simulink model "navigator"  (R2013b)
settings: Solver=FixedStepDiscrete  StartTime=0.0  StopTime=inf  FixedStep=0.1  RelTol=1e-3
undefined symbols (not defined in the file): Earth, WGS84
libraries: aerolibtransform2 x3, simulink_extras x2
settings Model: Creator=Matteo  LastModifiedBy=Gianluca Rossetti
settings OptimizationCC: OptimizeModelRefInitCode=on  LifeSpan=Inf
settings HardwareCC: ProdBitPerInt=16  ProdBitPerPointer=8  ProdIntDivRoundTo=Zero  ProdEndianess=LittleEndian  ProdWordSize=8  ProdHWDeviceType=Atmel->AVR
settings RTWCC: SystemTargetFile=ert.tlc  GenCodeOnly=on  TemplateMakefile=ert_default_tmf  Description=Embedded Coder  ProcessScript=ert_make_rtw_hook  BuildConfiguration=Faster Runs  TargetLang=C++  CheckMdlBeforeBuild=Warning
settings CodeAppCC: IgnoreCustomStorageClasses=off
settings ERTTargetCC: CodeReplacementLibrary=ANSI_C  GenerateSampleERTMain=on  ERTCustomFileTemplate=example_file_process.tlc

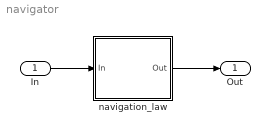
== system navigator ==
  In : Inport  OutDataTypeStr=single  PortDimensions=16
  navigation_law : Subsystem
  Out : Outport  OutDataTypeStr=single  PortDimensions=8
  wires:
  In/1 -> navigation_law/1(In)
  navigation_law/1(Out) -> Out/1

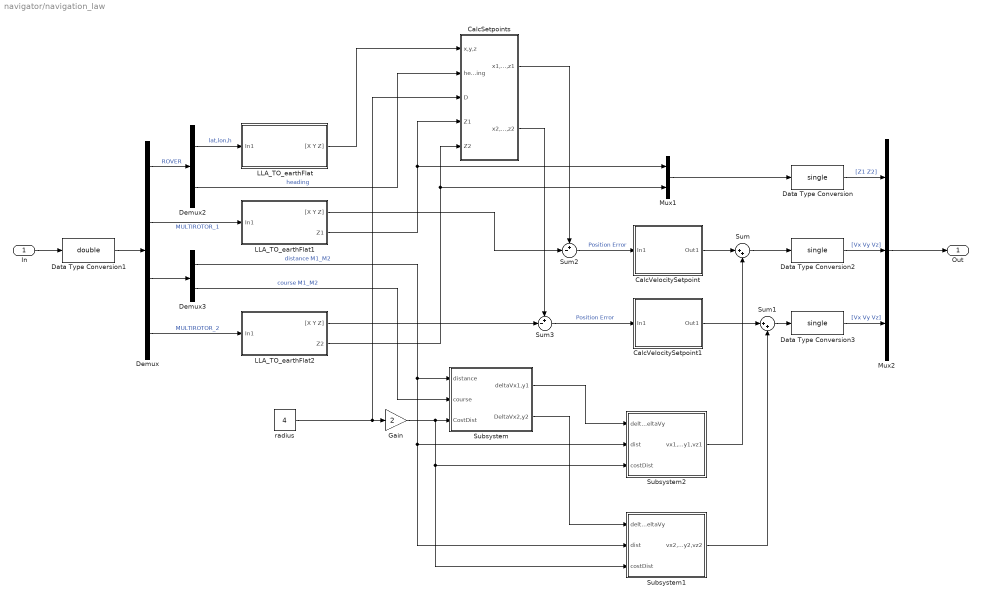
== system navigator/navigation_law ==
  In : Inport
  CalcSetpoints : Subsystem
  CalcVelocitySetpoint : Subsystem
  CalcVelocitySetpoint1 : Subsystem
  Data Type Conversion : DataTypeConversion  OutDataTypeStr=single
  Data Type Conversion1 : DataTypeConversion  OutDataTypeStr=double
  Data Type Conversion2 : DataTypeConversion  OutDataTypeStr=single
  Data Type Conversion3 : DataTypeConversion  OutDataTypeStr=single
  Demux : Demux  Outputs=[4 5 2 5]
  Demux2 : Demux  Outputs=[3 1]
  Demux3 : Demux  Outputs=2
  Gain : Gain  Gain=2
  LLA_TO_earthFlat : Subsystem
  LLA_TO_earthFlat1 : Subsystem
  LLA_TO_earthFlat2 : Subsystem
  Mux1 : Mux  Inputs=[1 1]
  Mux2 : Mux  Inputs=[2 3 3]
  Subsystem : Subsystem
  Subsystem1 : Subsystem
  Subsystem2 : Subsystem
  Sum : Sum  Inputs=|++
  Sum1 : Sum  Inputs=|++
  Sum2 : Sum  Inputs=+-|
  Sum3 : Sum  Inputs=+-|
  radius : Constant  Value=4
  Out : Outport
  wires:
  Demux/1 -> Demux2/1  "ROVER"
  Demux/4 -> LLA_TO_earthFlat2/1(In1)  "MULTIROTOR_2"
  Data Type Conversion/1 -> Mux2/1  "[Z1 Z2]"
  In/1 -> Data Type Conversion1/1
  Data Type Conversion1/1 -> Demux/1
  Mux2/1 -> Out/1
  Demux/2 -> LLA_TO_earthFlat1/1(In1)  "MULTIROTOR_1"
  LLA_TO_earthFlat1/1("[X Y Z]") -> Sum2/2
  Data Type Conversion2/1 -> Mux2/2  "[Vx Vy Vz]"
  Sum2/1 -> CalcVelocitySetpoint/1(In1)  "Position Error"
  CalcVelocitySetpoint/1(Out1) -> Sum/1
  LLA_TO_earthFlat2/1("[X Y Z]") -> Sum3/2
  Sum3/1 -> CalcVelocitySetpoint1/1(In1)  "Position Error"
  CalcVelocitySetpoint1/1(Out1) -> Sum1/1
  Data Type Conversion3/1 -> Mux2/3  "[Vx Vy Vz]"
  Demux2/1 -> LLA_TO_earthFlat/1(In1)  "lat,lon,h"
  LLA_TO_earthFlat/1("[X Y Z]") -> CalcSetpoints/1(x,y,z)
  Demux2/2 -> CalcSetpoints/2(heading)  "heading"
  CalcSetpoints/1(x1,y1,z1) -> Sum2/1
  CalcSetpoints/2(x2,y2,z2) -> Sum3/1
  radius/1 -> Gain/1, CalcSetpoints/3(D)
  LLA_TO_earthFlat1/2(Z1) -> Mux1/1, CalcSetpoints/4(Z1)
  LLA_TO_earthFlat2/2(Z2) -> CalcSetpoints/5(Z2), Mux1/2
  Demux/3 -> Demux3/1
  Demux3/1 -> Subsystem1/2(dist), Subsystem2/2(dist), Subsystem/1(distance)  "distance M1_M2"
  Sum/1 -> Data Type Conversion2/1
  Sum1/1 -> Data Type Conversion3/1
  Subsystem/1(deltaVx1,y1) -> Subsystem2/1("deltaVx, deltaVy")
  Mux1/1 -> Data Type Conversion/1
  Demux3/2 -> Subsystem/2(course)  "course M1_M2"
  Subsystem/2(DeltaVx2,y2) -> Subsystem1/1("deltaVx, deltaVy")
  Subsystem1/1(vx2,vy2,vz2) -> Sum1/2
  Subsystem2/1(vx1,vy1,vz1) -> Sum/2
  Gain/1 -> Subsystem1/3(costDist), Subsystem2/3(costDist), Subsystem/3(CostDist)

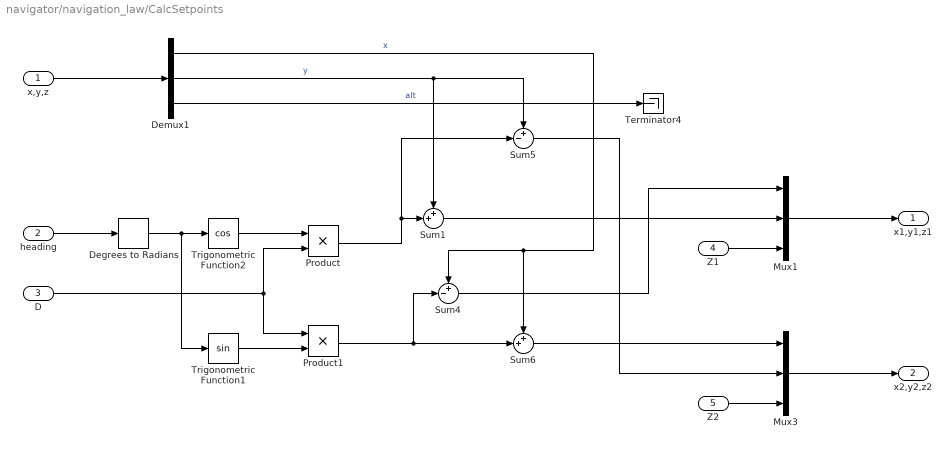
== system navigator/navigation_law/CalcSetpoints ==
  x,y,z : Inport
  heading : Inport  Port=2
  D : Inport  Port=3
  Z1 : Inport  Port=4
  Z2 : Inport  Port=5
  Degrees to Radians : simulink_extras/Transformations/Degrees to Radians
  Demux1 : Demux  Outputs=[1 1 1]
  Mux1 : Mux  Inputs=[1 1 1]
  Mux3 : Mux  Inputs=[1 1 1]
  Product : Product
  Product1 : Product
  Sum1 : Sum  Inputs=++|
  Sum4 : Sum  Inputs=+-|
  Sum5 : Sum  Inputs=+-|
  Sum6 : Sum  Inputs=++|
  Terminator4 : Terminator
  Trigonometric Function1 : Trigonometry
  Trigonometric Function2 : Trigonometry  Operator=cos
  x1,y1,z1 : Outport
  x2,y2,z2 : Outport  Port=2
  wires:
  Sum5/1 -> Mux3/2
  Sum6/1 -> Mux3/1
  Mux3/1 -> x2,y2,z2/1
  Demux1/1 -> Sum4/1, Sum6/1  "x"
  Mux1/1 -> x1,y1,z1/1
  Sum4/1 -> Mux1/1
  Product1/1 -> Sum6/2, Sum4/2
  heading/1 -> Degrees to Radians/1
  Demux1/2 -> Sum5/1, Sum1/1  "y"
  Sum1/1 -> Mux1/2
  Demux1/3 -> Terminator4/1  "alt"
  Product/1 -> Sum5/2, Sum1/2
  D/1 -> Product1/1, Product/2
  x,y,z/1 -> Demux1/1
  Degrees to Radians/1 -> Trigonometric Function1/1, Trigonometric Function2/1
  Trigonometric Function2/1 -> Product/1
  Trigonometric Function1/1 -> Product1/2
  Z2/1 -> Mux3/3
  Z1/1 -> Mux1/3

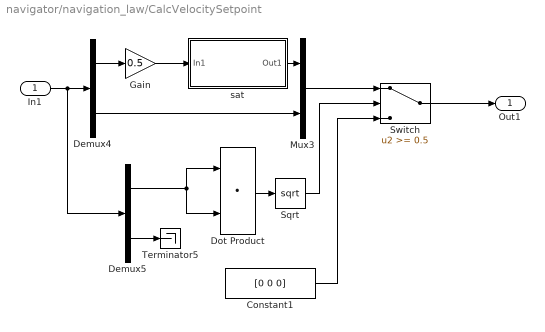
== system navigator/navigation_law/CalcVelocitySetpoint ==
  In1 : Inport
  Constant1 : Constant  Value=[0 0 0]
  Demux4 : Demux  Outputs=[2 1]
  Demux5 : Demux  Outputs=[2 1]
  Dot Product : DotProduct  InputSameDT=on  OutDataTypeStr=Inherit: Inherit via internal rule
  Gain : Gain  Gain=0.5
  Mux3 : Mux  Inputs=[2 1]
  Sqrt : Sqrt  SaturateOnIntegerOverflow=on
  Switch : Switch  Threshold=0.5
  Terminator5 : Terminator
  "sat " : Subsystem  mask{k_sat=5}
      mask prompts: k_sat "Saturatore"
  Out1 : Outport
  wires:
  In1/1 -> Demux4/1, Demux5/1
  Demux4/1 -> Gain/1
  "sat "/1(Out1) -> Mux3/1
  Demux4/2 -> Mux3/2
  Demux5/1 -> Dot Product/1, Dot Product/2
  Dot Product/1 -> Sqrt/1
  Demux5/2 -> Terminator5/1
  Sqrt/1 -> Switch/2
  Mux3/1 -> Switch/1
  Constant1/1 -> Switch/3
  Switch/1 -> Out1/1
  Gain/1 -> "sat "/1(In1)

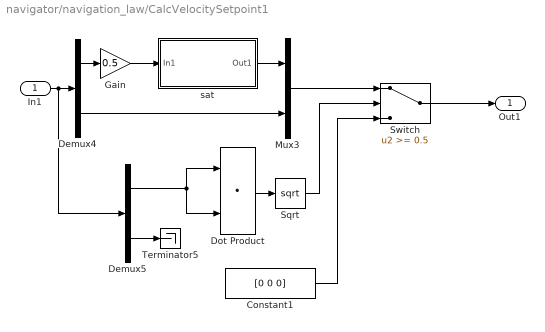
== system navigator/navigation_law/CalcVelocitySetpoint1 ==
  In1 : Inport
  Constant1 : Constant  Value=[0 0 0]
  Demux4 : Demux  Outputs=[2 1]
  Demux5 : Demux  Outputs=[2 1]
  Dot Product : DotProduct  InputSameDT=on  OutDataTypeStr=Inherit: Inherit via internal rule
  Gain : Gain  Gain=0.5
  Mux3 : Mux  Inputs=[2 1]
  Sqrt : Sqrt  SaturateOnIntegerOverflow=on
  Switch : Switch  Threshold=0.5
  Terminator5 : Terminator
  "sat " : Subsystem  mask{k_sat=5}
      mask prompts: k_sat "Saturatore"
  Out1 : Outport
  wires:
  Switch/1 -> Out1/1
  Constant1/1 -> Switch/3
  Mux3/1 -> Switch/1
  Sqrt/1 -> Switch/2
  Demux5/2 -> Terminator5/1
  Dot Product/1 -> Sqrt/1
  Demux5/1 -> Dot Product/2, Dot Product/1
  Demux4/2 -> Mux3/2
  "sat "/1(Out1) -> Mux3/1
  Demux4/1 -> Gain/1
  In1/1 -> Demux4/1, Demux5/1
  Gain/1 -> "sat "/1(In1)

== system navigator/navigation_law/LLA_TO_earthFlat ==
  In1 : Inport
  Constant : Constant  Value=0  OutDataTypeStr=single
  Demux1 : Demux  Outputs=[2 1]
  LLA to Flat Earth : aerolibtransform2/LLA to Flat Earth  units=Metric (MKS)  ptype=Earth (WGS84)  F=1/298.257223563  R=6378137  LL0="[44.201892800000003  12.062565800000000]"  psi=0
  "[X Y Z]" : Outport
  wires:
  Constant/1 -> LLA to Flat Earth/3
  Demux1/1 -> LLA to Flat Earth/1
  LLA to Flat Earth/1 -> "[X Y Z]"/1  "earth_flat"
  Demux1/2 -> LLA to Flat Earth/2
  In1/1 -> Demux1/1

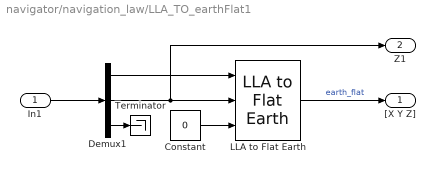
== system navigator/navigation_law/LLA_TO_earthFlat1 ==
  In1 : Inport
  Constant : Constant  Value=0  OutDataTypeStr=single
  Demux1 : Demux  Outputs=[2 1 2]
  LLA to Flat Earth : aerolibtransform2/LLA to Flat Earth  units=Metric (MKS)  ptype=Earth (WGS84)  F=1/298.257223563  R=6378137  LL0="[44.201892800000003  12.062565800000000]"  psi=0
  Terminator : Terminator
  "[X Y Z]" : Outport
  Z1 : Outport  Port=2
  wires:
  Demux1/3 -> Terminator/1
  In1/1 -> Demux1/1
  Demux1/2 -> Z1/1, LLA to Flat Earth/2
  LLA to Flat Earth/1 -> "[X Y Z]"/1  "earth_flat"
  Demux1/1 -> LLA to Flat Earth/1
  Constant/1 -> LLA to Flat Earth/3

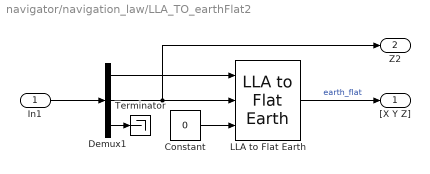
== system navigator/navigation_law/LLA_TO_earthFlat2 ==
  In1 : Inport
  Constant : Constant  Value=0  OutDataTypeStr=single
  Demux1 : Demux  Outputs=[2 1 2]
  LLA to Flat Earth : aerolibtransform2/LLA to Flat Earth  units=Metric (MKS)  ptype=Earth (WGS84)  F=1/298.257223563  R=6378137  LL0="[44.201892800000003  12.062565800000000]"  psi=0
  Terminator : Terminator
  "[X Y Z]" : Outport
  Z2 : Outport  Port=2
  wires:
  Constant/1 -> LLA to Flat Earth/3
  Demux1/1 -> LLA to Flat Earth/1
  LLA to Flat Earth/1 -> "[X Y Z]"/1  "earth_flat"
  Demux1/2 -> Z2/1, LLA to Flat Earth/2
  In1/1 -> Demux1/1
  Demux1/3 -> Terminator/1

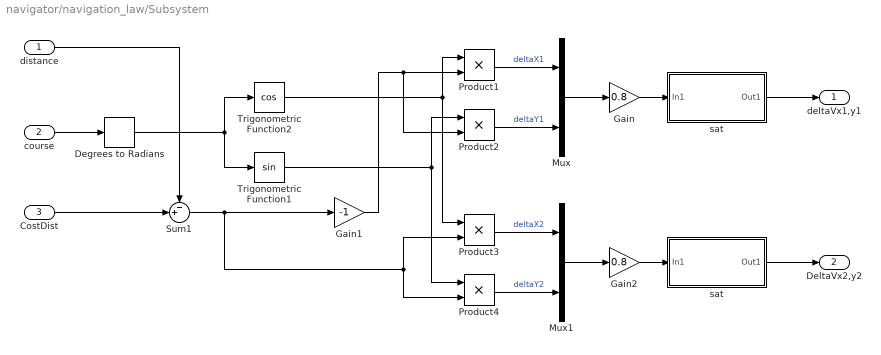
== system navigator/navigation_law/Subsystem ==
  distance : Inport
  course : Inport  Port=2
  CostDist : Inport  Port=3
  Degrees to Radians : simulink_extras/Transformations/Degrees to Radians
  Gain : Gain  Gain=0.8
  Gain1 : Gain  Gain=-1
  Gain2 : Gain  Gain=0.8
  Mux : Mux  Inputs=2
  Mux1 : Mux  Inputs=2
  Product{1..4} (4 alike) : Product
  Sum1 : Sum  Inputs=-+|
  Trigonometric Function1 : Trigonometry
  Trigonometric Function2 : Trigonometry  Operator=cos
  "sat " : Subsystem  mask{k_sat=3}
      mask prompts: k_sat "Saturatore"
  "sat " : Subsystem  mask{k_sat=3}
      mask prompts: k_sat "Saturatore"
  deltaVx1,y1 : Outport
  DeltaVx2,y2 : Outport  Port=2
  wires:
  Product2/1 -> Mux/2  "deltaY1"
  Product1/1 -> Mux/1  "deltaX1"
  Sum1/1 -> Product3/2, Product4/2, Gain1/1
  Gain/1 -> "sat "/1(In1)
  Product3/1 -> Mux1/1  "deltaX2"
  "sat "/1(Out1) -> DeltaVx2,y2/1
  Gain1/1 -> Product2/2, Product1/2
  Mux/1 -> Gain/1
  Trigonometric Function2/1 -> Product1/1, Product3/1
  Degrees to Radians/1 -> Trigonometric Function2/1, Trigonometric Function1/1
  distance/1 -> Sum1/1
  "sat "/1(Out1) -> deltaVx1,y1/1
  Gain2/1 -> "sat "/1(In1)
  course/1 -> Degrees to Radians/1
  Mux1/1 -> Gain2/1
  Trigonometric Function1/1 -> Product2/1, Product4/1
  Product4/1 -> Mux1/2  "deltaY2"
  CostDist/1 -> Sum1/2

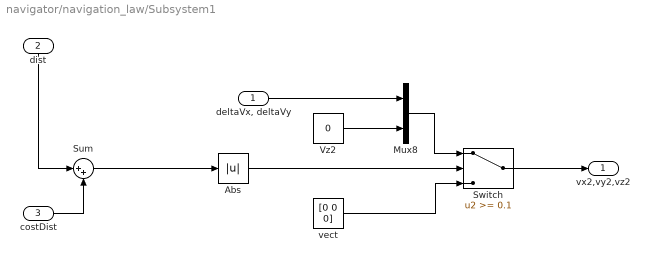
== system navigator/navigation_law/Subsystem1 ==
  "deltaVx, deltaVy" : Inport
  dist : Inport  Port=2
  costDist : Inport  Port=3
  Abs : Abs
  Mux8 : Mux  Inputs=[2 1]
  Sum : Sum  Inputs=|++
  Switch : Switch  Threshold=0.1
  Vz2 : Constant  Value=0
  vect : Constant  Value=[0 0 0]
  vx2,vy2,vz2 : Outport
  wires:
  "deltaVx, deltaVy"/1 -> Mux8/1
  Vz2/1 -> Mux8/2
  Mux8/1 -> Switch/1
  Switch/1 -> vx2,vy2,vz2/1
  vect/1 -> Switch/3
  dist/1 -> Sum/1
  costDist/1 -> Sum/2
  Sum/1 -> Abs/1
  Abs/1 -> Switch/2

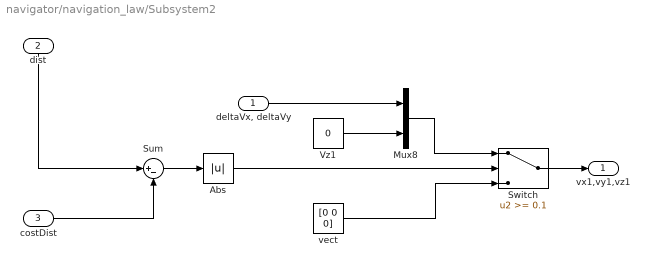
== system navigator/navigation_law/Subsystem2 ==
  "deltaVx, deltaVy" : Inport
  dist : Inport  Port=2
  costDist : Inport  Port=3
  Abs : Abs
  Mux8 : Mux  Inputs=[2 1]
  Sum : Sum  Inputs=|+-
  Switch : Switch  Threshold=0.1
  Vz1 : Constant  Value=0
  vect : Constant  Value=[0 0 0]
  vx1,vy1,vz1 : Outport
  wires:
  dist/1 -> Sum/1
  vect/1 -> Switch/3
  Switch/1 -> vx1,vy1,vz1/1
  Mux8/1 -> Switch/1
  Vz1/1 -> Mux8/2
  "deltaVx, deltaVy"/1 -> Mux8/1
  costDist/1 -> Sum/2
  Sum/1 -> Abs/1
  Abs/1 -> Switch/2

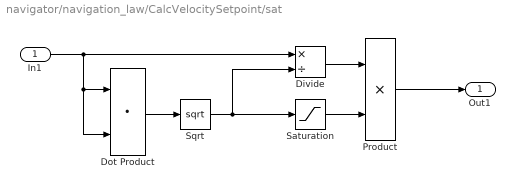
== system navigator/navigation_law/CalcVelocitySetpoint/sat  ==
  In1 : Inport
  Divide : Product  Inputs=*/
  Dot Product : DotProduct  InputSameDT=on  OutDataTypeStr=Inherit: Inherit via internal rule
  Product : Product
  Saturation : Saturate  UpperLimit=k_sat  LowerLimit=0
  Sqrt : Sqrt  SaturateOnIntegerOverflow=on
  Out1 : Outport
  wires:
  Divide/1 -> Product/1
  Product/1 -> Out1/1
  Sqrt/1 -> Divide/2, Saturation/1
  In1/1 -> Divide/1, Dot Product/1, Dot Product/2
  Dot Product/1 -> Sqrt/1
  Saturation/1 -> Product/2

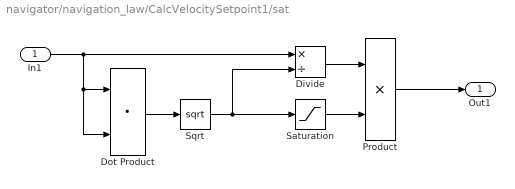
== system navigator/navigation_law/CalcVelocitySetpoint1/sat  ==
  In1 : Inport
  Divide : Product  Inputs=*/
  Dot Product : DotProduct  InputSameDT=on  OutDataTypeStr=Inherit: Inherit via internal rule
  Product : Product
  Saturation : Saturate  UpperLimit=k_sat  LowerLimit=0
  Sqrt : Sqrt  SaturateOnIntegerOverflow=on
  Out1 : Outport
  wires:
  Saturation/1 -> Product/2
  Dot Product/1 -> Sqrt/1
  In1/1 -> Dot Product/2, Dot Product/1, Divide/1
  Sqrt/1 -> Saturation/1, Divide/2
  Product/1 -> Out1/1
  Divide/1 -> Product/1

== system navigator/navigation_law/Subsystem/sat  ==
  In1 : Inport
  Divide : Product  Inputs=*/
  Dot Product : DotProduct  InputSameDT=on  OutDataTypeStr=Inherit: Inherit via internal rule
  Product : Product
  Saturation : Saturate  UpperLimit=k_sat  LowerLimit=0
  Sqrt : Sqrt  SaturateOnIntegerOverflow=on
  Out1 : Outport
  wires:
  Saturation/1 -> Product/2
  Dot Product/1 -> Sqrt/1
  In1/1 -> Dot Product/2, Dot Product/1, Divide/1
  Sqrt/1 -> Saturation/1, Divide/2
  Product/1 -> Out1/1
  Divide/1 -> Product/1

== system navigator/navigation_law/Subsystem/sat  ==
  In1 : Inport
  Divide : Product  Inputs=*/
  Dot Product : DotProduct  InputSameDT=on  OutDataTypeStr=Inherit: Inherit via internal rule
  Product : Product
  Saturation : Saturate  UpperLimit=k_sat  LowerLimit=0
  Sqrt : Sqrt  SaturateOnIntegerOverflow=on
  Out1 : Outport
  wires:
  Divide/1 -> Product/1
  Product/1 -> Out1/1
  Sqrt/1 -> Divide/2, Saturation/1
  In1/1 -> Divide/1, Dot Product/1, Dot Product/2
  Dot Product/1 -> Sqrt/1
  Saturation/1 -> Product/2
